simulink model "mfcnreset_periodic1"  (Simulink 6.3)
settings: Solver=FixedStepDiscrete  StartTime=0.0  StopTime=10.0  FixedStep=0.1  RelTol=1e-3
undefined symbols (not defined in the file or in its folder): DiscIntNeverNeededParam
settings Model: Creator=matthewe  LastModifiedBy=tsimsek  ExtModeEnableOpenProtocolUploading=on  ExtModeOpenProtocolUploadingEqualLengthVectors=off  ExtModeAutoUpdateStatusClock=off  StrictBusMsg=None
settings DataIOCC: SignalLogging=off  SignalLoggingName=sigsOut
settings OptimizationCC: LifeSpan=1
settings DebuggingCC: SolverPrmCheckMsg=none  InheritedTsInSrcMsg=none
settings RTWCC: SystemTargetFile=ert.tlc  TemplateMakefile=ert_default_tmf  Description=Real-Time Workshop Embedded Coder (no auto configuration)  ProcessScript=ert_make_rtw_hook
settings CodeAppCC: IgnoreCustomStorageClasses=off
settings ERTTargetCC: TargetFcnLib=ansi_tfl_tmw.mat  GenFloatMathFcnCalls=ANSI_C  GenerateSampleERTMain=on  InlinedParameterPlacement=NonHierarchical  ERTCustomFileTemplate=example_file_process.tlc  InitialValueSource=Model

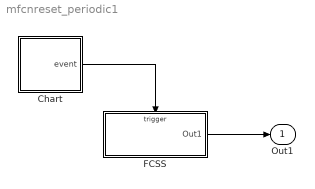
== system mfcnreset_periodic1 ==
  Chart : Stateflow chart
  FCSS : Subsystem  TreatAsAtomicUnit=on
  Out1 : Outport
  wires:
  Chart/1(event) -> FCSS/Trigger
  FCSS/1(Out1) -> Out1/1

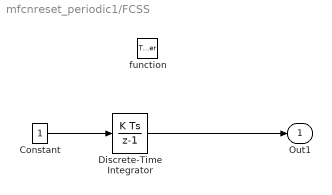
== system mfcnreset_periodic1/FCSS ==
  function : TriggerPort  TriggerType=function-call  StatesWhenEnabling=reset  SampleTimeType=periodic  SampleTime=0.1
  Constant : Constant
  Discrete-Time Integrator : DiscreteIntegrator  InitialCondition=2  SampleTime=-1  ICPrevOutput=DiscIntNeverNeededParam  ICPrevScaledInput=DiscIntNeverNeededParam
  Out1 : Outport  OutputWhenDisabled=reset  InitialOutput=1
  wires:
  Discrete-Time Integrator/1 -> Out1/1
  Constant/1 -> Discrete-Time Integrator/1

== stateflow chart Chart ==
  state A
  state B
    bind: event
    B -> (junction 5) [order 1]
    (default) -> (junction 5)
    (junction 5) -> (junction 6) : {event;}
  A -> B : [every(10,tick)]
  B -> A [order 1] : [every(10,tick)]
  (default) -> A
  events: event output FUNCTION_CALL_EVENT
